simulink model "Testbench_030226"  (R2025b)
settings: Solver=FixedStepDiscrete  StartTime=0.0  StopTime=size(bit_seq, 2) * 1E-3  RelTol=1e-3
InitFcn:
  | bit_seq = [0 0 0 1 0 0 1 0 0 1];
libraries: hdlsllib x2, simulink x1, dspswit3 x1
settings Model: DataTypeOverride=Off  Creator=abstract  LastModifiedBy=abstract
settings OptimizationCC: BlockReduction=off  ConditionallyExecuteInputs=off  DefaultParameterBehavior=Inlined  InheritOutputTypeSmallerThanSingle=on
settings DebuggingCC: AlgebraicLoopMsg=error  SingleTaskRateTransMsg=error  UnconnectedInputMsg=warning  UnconnectedOutputMsg=warning  UnconnectedLineMsg=warning
settings HardwareCC: ProdBitPerPointer=32.0  ProdBitPerSizeT=32.0  ProdBitPerPtrDiffT=32.0  ProdLargestAtomicFloat=None  ProdIntDivRoundTo=Undefined  ProdEndianess=Unspecified  ProdWordSize=32.0  ProdHWDeviceType=ASIC/FPGA->ASIC/FPGA  TargetBitPerLong=64.0  TargetBitPerPointer=64.0  TargetBitPerSizeT=64.0  TargetBitPerPtrDiffT=64.0  TargetLongLongMode=on  TargetIntDivRoundTo=Zero  TargetEndianess=LittleEndian  TargetWordSize=64.0  TargetHWDeviceType=Custom Processor->MATLAB Host Computer  ProdEqTarget=off

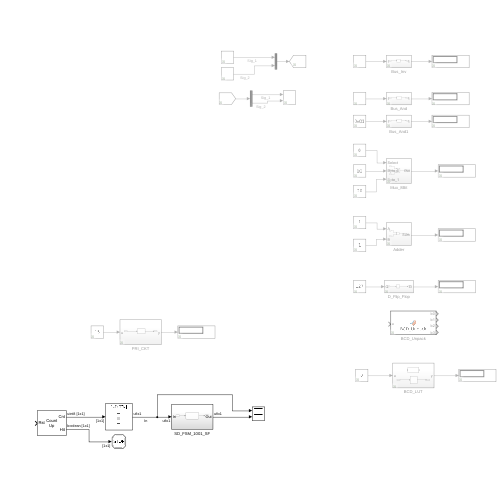
[thumbnail: Simulink's stored preview of the top-level diagram]
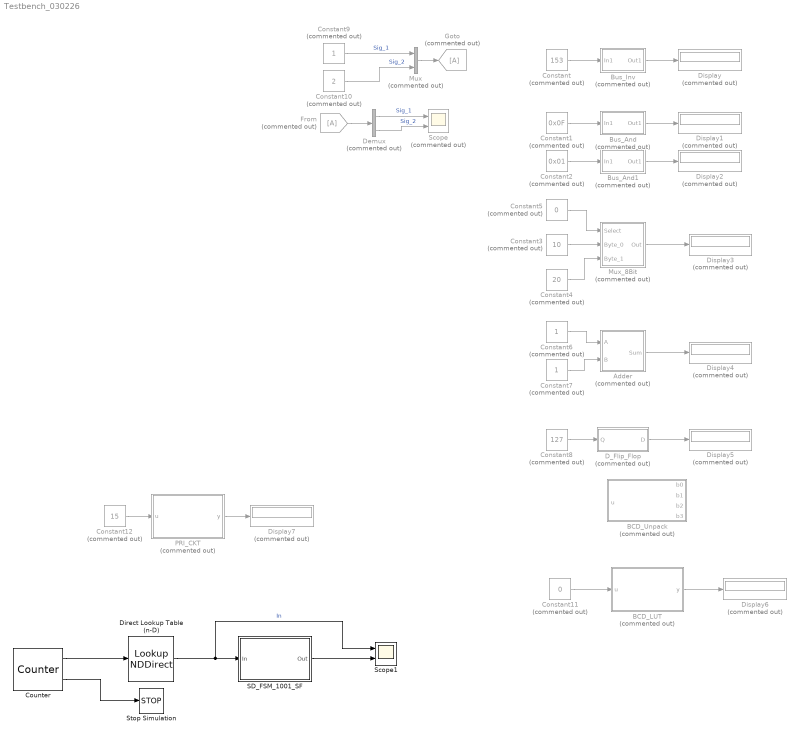
== system Testbench_030226 ==
  Adder : Subsystem  Commented=on
  BCD_LUT : Subsystem  Commented=on
  BCD_Unpack : MATLAB Function  Commented=on  TreatAsAtomicUnit=on
  Bus_And : Subsystem  Commented=on
  Bus_And1 : Subsystem  Commented=on
  Bus_Inv : Subsystem  Commented=on
  Constant : Constant  Commented=on  Value=153  OutDataTypeStr=Inherit: Inherit via back propagation  SampleTime=-1
  Constant1 : Constant  Commented=on  Value=0x0F  OutDataTypeStr=Inherit: Inherit via back propagation  SampleTime=-1
  Constant10 : Constant  Commented=on  Value=2  SampleTime=-1
  Constant11 : Constant  Commented=on  Value=0  OutDataTypeStr=Inherit: Inherit via back propagation  SampleTime=-1
  Constant12 : Constant  Commented=on  Value=15  OutDataTypeStr=Inherit: Inherit via back propagation  SampleTime=-1
  Constant2 : Constant  Commented=on  Value=0x01  OutDataTypeStr=Inherit: Inherit via back propagation  SampleTime=-1
  Constant3 : Constant  Commented=on  Value=10  OutDataTypeStr=Inherit: Inherit via back propagation  SampleTime=-1
  Constant4 : Constant  Commented=on  Value=20  OutDataTypeStr=Inherit: Inherit via back propagation  SampleTime=-1
  Constant5 : Constant  Commented=on  Value=0  OutDataTypeStr=Inherit: Inherit via back propagation  SampleTime=-1
  Constant6 : Constant  Commented=on  OutDataTypeStr=Inherit: Inherit via back propagation  SampleTime=-1
  Constant7 : Constant  Commented=on  OutDataTypeStr=Inherit: Inherit via back propagation  SampleTime=-1
  Constant8 : Constant  Commented=on  Value=127  OutDataTypeStr=Inherit: Inherit via back propagation  SampleTime=-1
  Constant9 : Constant  Commented=on  SampleTime=-1
  Counter : dspswit3/Counter  Direction=Up  CountEvent=Free running  CounterSize=User defined  MaxCount=size(bit_seq, 2) - 1  InitialCount=0  Output=Count and Hit  HitValue=size(bit_seq, 2) - 1  ResetInput=on  SamplesPerFrame=1  Ts=-1  CntDtype=uint8  HitDtype=Logical
  D_Flip_Flop : Subsystem  Commented=on
  Demux : Demux  Commented=on  Outputs=2
  Direct Lookup Table (n-D) : LookupNDDirect  NumberOfTableDimensions=1  Table=bit_seq  TableDataTypeStr=fixdt(0,1,0)
  Display{,1..7} (8 alike) : Display  Commented=on
  From : From  Commented=on
  Goto : Goto  Commented=on
  Mux : Mux  Commented=on  Inputs=2
  Mux_8Bit : Subsystem  Commented=on
  PRI_CKT : Subsystem  Commented=on
  SD_FSM_1001_SF : Subsystem
  Scope : Scope  Commented=on  NumInputPorts=2
      settings: ActiveDisplayYMinimum=-1  ActiveDisplayYMaximum=1
  Scope1 : Scope  NumInputPorts=2
      settings: ActiveDisplayYMinimum=-0.12499999999999997  ActiveDisplayYMaximum=1.125
  Stop Simulation : Stop
  wires:
  Constant/1 -> Bus_Inv/1(In1)
  Bus_Inv/1(Out1) -> Display/1
  Bus_And/1(Out1) -> Display1/1
  Bus_And1/1(Out1) -> Display2/1
  Constant1/1 -> Bus_And/1(In1)
  Constant2/1 -> Bus_And1/1(In1)
  Constant5/1 -> Mux_8Bit/1(Select)
  Constant3/1 -> Mux_8Bit/2(Byte_0)
  Constant4/1 -> Mux_8Bit/3(Byte_1)
  Mux_8Bit/1(Out) -> Display3/1
  Constant6/1 -> Adder/1(A)
  Constant7/1 -> Adder/2(B)
  Adder/1(Sum) -> Display4/1
  Constant8/1 -> D_Flip_Flop/1(Q)
  D_Flip_Flop/1(D) -> Display5/1
  Constant9/1 -> Mux/1  "Sig_1"
  Constant10/1 -> Mux/2  "Sig_2"
  Mux/1 -> Goto/1
  From/1 -> Demux/1
  Demux/1 -> Scope/1  "Sig_1"
  Demux/2 -> Scope/2  "Sig_2"
  Constant11/1 -> BCD_LUT/1(u)
  BCD_LUT/1(y) -> Display6/1
  Constant12/1 -> PRI_CKT/1(u)
  PRI_CKT/1(y) -> Display7/1
  Counter/2 -> Stop Simulation/1
  Direct Lookup Table (n-D)/1 -> SD_FSM_1001_SF/1(In), Scope1/1  "In"
  Counter/1 -> Direct Lookup Table (n-D)/1
  SD_FSM_1001_SF/1(Out) -> Scope1/2

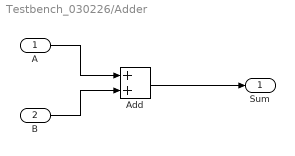
== system Testbench_030226/Adder ==
  A : Inport  OutDataTypeStr=fixdt(0,1,0)
  B : Inport  Port=2  OutDataTypeStr=fixdt(0,1,0)
  Add : Sum  OutDataTypeStr=fixdt(0,1,0)
  Sum : Outport  OutDataTypeStr=fixdt(0,1,0)
  wires:
  B/1 -> Add/2
  A/1 -> Add/1
  Add/1 -> Sum/1

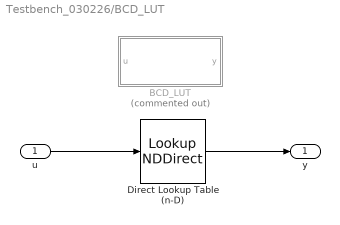
== system Testbench_030226/BCD_LUT ==
  u : Inport  OutDataTypeStr=fixdt(0,2,0)
  BCD_LUT : MATLAB Function  Commented=on  TreatAsAtomicUnit=on
  Direct Lookup Table (n-D) : LookupNDDirect  NumberOfTableDimensions=1  Table=[fi(0b1111110, 0, 7, 0), fi(0b0110000, 0, 7, 0), fi(0b1101101, 0, 7, 0), fi(0b1111001, 0, 7, 0)]
  y : Outport  OutDataTypeStr=fixdt(0,7,0)
  wires:
  u/1 -> Direct Lookup Table (n-D)/1
  Direct Lookup Table (n-D)/1 -> y/1

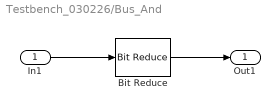
== system Testbench_030226/Bus_And ==
  In1 : Inport  OutDataTypeStr=fixdt(0,4,0)
  Bit Reduce : hdlsllib/Logic and Bit Operations/Bit Reduce  mode=AND
  Out1 : Outport  OutDataTypeStr=fixdt(0,1,0)
  wires:
  In1/1 -> Bit Reduce/1
  Bit Reduce/1 -> Out1/1

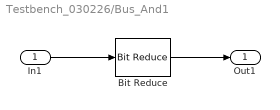
== system Testbench_030226/Bus_And1 ==
  In1 : Inport  OutDataTypeStr=fixdt(0,4,0)
  Bit Reduce : hdlsllib/Logic and Bit Operations/Bit Reduce  mode=AND
  Out1 : Outport  OutDataTypeStr=fixdt(0,1,0)
  wires:
  In1/1 -> Bit Reduce/1
  Bit Reduce/1 -> Out1/1

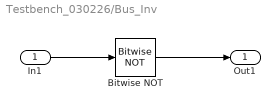
== system Testbench_030226/Bus_Inv ==
  In1 : Inport  OutDataTypeStr=fixdt(0,8,0)
  Bitwise NOT : simulink/Logic and Bit Operations/Bitwise Operator  logicop=NOT  UseBitMask=off  BitMask=bin2dec('11011001')  BitMaskRealWorld=Stored Integer
      settings: LibrarySourceBlock=|
      | simulink/Quick Insert/Logic and Bit
      | Operations/Bitwise NOT
  Out1 : Outport  OutDataTypeStr=fixdt(0,8,0)
  wires:
  In1/1 -> Bitwise NOT/1
  Bitwise NOT/1 -> Out1/1

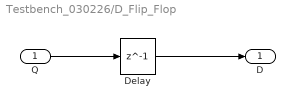
== system Testbench_030226/D_Flip_Flop ==
  Q : Inport  OutDataTypeStr=uint8
  Delay : Delay  DelayLength=1  InputProcessing=Columns as channels (frame based)
  D : Outport  OutDataTypeStr=uint8
  wires:
  Q/1 -> Delay/1
  Delay/1 -> D/1

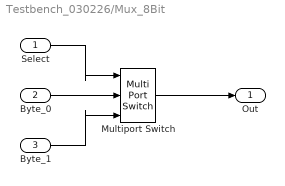
== system Testbench_030226/Mux_8Bit ==
  Select : Inport  OutDataTypeStr=fixdt(0,1,0)
  Byte_0 : Inport  Port=2  OutDataTypeStr=uint8
  Byte_1 : Inport  Port=3  OutDataTypeStr=uint8
  Multiport Switch : MultiPortSwitch  DataPortOrder=Zero-based contiguous  Inputs=2  zeroidx=on  SaturateOnIntegerOverflow=off  InputSameDT=off
  Out : Outport
  wires:
  Byte_0/1 -> Multiport Switch/2
  Select/1 -> Multiport Switch/1
  Byte_1/1 -> Multiport Switch/3
  Multiport Switch/1 -> Out/1

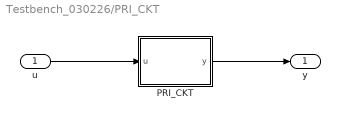
== system Testbench_030226/PRI_CKT ==
  u : Inport  OutDataTypeStr=fixdt(0,4,0)
  PRI_CKT : MATLAB Function  TreatAsAtomicUnit=on
  y : Outport  OutDataTypeStr=fixdt(0,4,0)
  wires:
  u/1 -> PRI_CKT/1(u)
  PRI_CKT/1(y) -> y/1

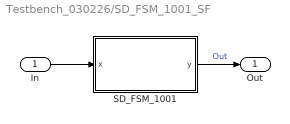
== system Testbench_030226/SD_FSM_1001_SF ==
  In : Inport  OutDataTypeStr=fixdt(0,1,0)
  SD_FSM_1001 : Stateflow chart  TreatAsAtomicUnit=on
  Out : Outport  OutDataTypeStr=fixdt(0,1,0)
  wires:
  SD_FSM_1001/1(y) -> Out/1  "Out"
  In/1 -> SD_FSM_1001/1(x)

== matlab function Testbench_030226/BCD_LUT/BCD_LUT ==
  data: u input; y output
function y = BCD_LUT(u)

bcd_lut = fi([ ...
    0b1111110,...
    0b0110000,...
    0b1101101,...
    0b1111001,...
    ], 0, 7, 0);

% switch u
%     case 0
%         y = fi(0b1111110, 0, 7, 0);
%     case 1
%         y = fi(0b0110000, 0, 7, 0);
%     case 2
%         y = fi(0b1101101, 0, 7, 0);
%     case 3
%         y = fi(0b1111001, 0, 7, 0);
%     case 4
%         y = fi(0b0110011, 0, 7, 0);
%     case 5
%         y = fi(0b1011011, 0, 7, 0);
%     case 6
%         y = fi(0b1011111, 0, 7, 0);
%     case 7
%         y = fi(0b1110000, 0, 7, 0);
%     case 8
%         y = fi(0b1111111, 0, 7, 0);
%     case 9
%         y = fi(0b1110011, 0, 7, 0);
%     otherwise
%         y = fi(0b0000000, 0, 7, 0);
% end

y = bcd_lut(u);

== matlab function Testbench_030226/BCD_Unpack ==
  data: u input; b0 output; b1 output; b2 output; b3 output
function [b0, b1, b2, b3] = BCD_Unpack(u)

b0 = bitget(u, 1);
b1 = bitget(u, 2);
b2 = bitget(u, 3);
b3 = bitget(u, 4);

== matlab function Testbench_030226/PRI_CKT/PRI_CKT ==
  data: u input; y output
function y = PRI_CKT(u)

if bitget(u, 4)
    y = fi(0b1000, 0, 4, 0);
elseif bitget(u, 3)
    y = fi(0b0100, 0, 4, 0);
elseif bitget(u, 2)
    y = fi(0b0010, 0, 4, 0);
elseif bitget(u, 1)
    y = fi(0b0001, 0, 4, 0);
else
    y = fi(0b0000, 0, 4, 0);
end

== stateflow chart Testbench_030226/SD_FSM_1001_SF/SD_FSM_1001 ==
  settings: stateMachineType=MOORE_MACHINE  executeAtInitialization=1
  state S__
    y = 0;
  state S_1
    y = 0;
  state S_10
    y = 0;
  state S_100
    y = 0;
  state S_1001
    y = 1;
  S_100 -> S__ [order 2] : [x == 0]
  (default) -> S__
  S__ -> S__ [order 1] : [x == 0]
  S_1 -> S_1 [order 1] : [x == 1]
  S__ -> S_1 [order 2] : [x == 1]
  S_1 -> S_10 [order 2] : [x == 0]
  S_10 -> S_100 [order 1] : [x == 0]
  S_1001 -> S_1 [order 2] : [x == 1]
  S_10 -> S_1 [order 2] : [x == 1]
  S_1001 -> S_10 [order 1] : [x == 0]
  S_100 -> S_1001 [order 1] : [x == 1]
  data: x input fixdt(0,1,0); y output fixdt(0,1,0)
